simulink model "scdpwm"  (Simulink 7.6)
settings: Solver=ode45  StartTime=0.0  StopTime=15  FixedStep=0.001  RelTol=1e-3
libraries: simulink x2, simulink_extras x1
settings Model: Creator=The MathWorks Inc.
settings OptimizationCC: InlineInvariantSignals=on  InitFltsAndDblsToZero=on
settings DebuggingCC: AlgebraicLoopMsg=none  SaveWithParameterizedLinksMsg=none  CheckExecutionContextPreStartOutputMsg=on  CheckExecutionContextRuntimeOutputMsg=on  SignalResolutionControl=TryResolveAllWithWarning  SolverPrmCheckMsg=none  MultiTaskDSMMsg=warning  MultiTaskCondExecSysMsg=none  UnconnectedInputMsg=none  UnconnectedOutputMsg=none  UnconnectedLineMsg=none  StrictBusMsg=None
settings RTWCC: IncludeERTFirstTime=on
settings GRTTargetCC: TargetFcnLib=ansi_tfl_tmw.mat

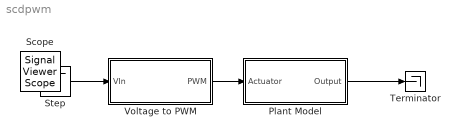
== system scdpwm ==
  Plant Model : Subsystem
  Step : Step  Before=0.4  After=0.4  SampleTime=0
  Terminator : Terminator
  Voltage to PWM : Subsystem
  Scope : SignalViewerScope  IOType=viewer  RefreshTime=0.035000
      settings: YMin=0.39  YMax=0.52
  wires:
  Voltage to PWM/1(PWM) -> Plant Model/1(Actuator)
  Plant Model/1(Output) -> Terminator/1
  Step/1 -> Voltage to PWM/1(VIn)

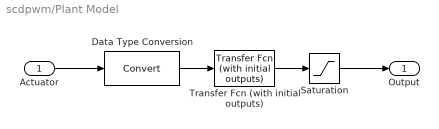
== system scdpwm/Plant Model ==
  Actuator : Inport
  Data Type Conversion : DataTypeConversion
  Saturation : Saturate  UpperLimit=inf  LowerLimit=-inf
  Transfer Fcn (with initial outputs) : simulink_extras/Additional Linear/Transfer Fcn (with initial outputs)  SystemSampleTime=-1  N=[1]  D="[1  1 1]"  Y0=0.4  U0=0.4
  Output : Outport
  wires:
  Actuator/1 -> Data Type Conversion/1
  Transfer Fcn (with initial outputs)/1 -> Saturation/1
  Saturation/1 -> Output/1
  Data Type Conversion/1 -> Transfer Fcn (with initial outputs)/1

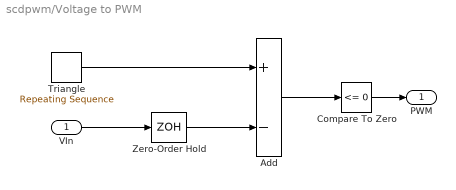
== system scdpwm/Voltage to PWM ==
  VIn : Inport
  Add : Sum  Inputs=+-  SampleTime=1/10000
  Compare To Zero : simulink/Logic and Bit Operations/Compare To Zero  SystemSampleTime=-1  relop=<=  LogicOutDataTypeMode=uint8
  Triangle : simulink/Sources/Repeating Sequence  SystemSampleTime=-1  rep_seq_t=[0 1/100/4 3/100/4 1/100]  rep_seq_y=[0.5 0 1 0.5]
  Zero-Order Hold : ZeroOrderHold  SampleTime=1/10000
  PWM : Outport
  wires:
  Triangle/1 -> Add/1
  VIn/1 -> Zero-Order Hold/1
  Add/1 -> Compare To Zero/1
  Compare To Zero/1 -> PWM/1
  Zero-Order Hold/1 -> Add/2
